simulink model "model_without_disturbance"  (R2015b)
settings: Solver=VariableStepAuto  StartTime=0.0  StopTime=5  RelTol=1e-3
values from neighbouring files (symbols this model uses):
  dg = [1 2 400]    [script.m]
  ng = 400    [script.m]
undefined symbols (not defined in the file or in its folder): denk, numk
settings Model: Creator=EriveltonDell  LastModifiedBy=EriveltonDell

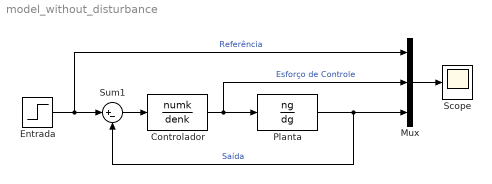
== system model_without_disturbance ==
  Controlador : TransferFcn  Numerator=numk  Denominator=denk
  Entrada : Step  SampleTime=0
  Mux : Mux  Inputs=3
  Planta : TransferFcn  Numerator=ng  Denominator=dg
  Scope : Scope
  Sum1 : Sum  Inputs=|+-
  wires:
  Controlador/1 -> Mux/2, Planta/1  "Esforço de Controle"
  Sum1/1 -> Controlador/1
  Entrada/1 -> Mux/1, Sum1/1  "Referência"
  Mux/1 -> Scope/1
  Planta/1 -> Mux/3, Sum1/2  "Saída"
